simulink model "Energy Domain TDPC Q2"  (R2021b)
settings: Solver=ode4  StartTime=0.0  StopTime=20  FixedStep=0.0001  RelTol=1e-3
libraries: slpidlib x2
settings Model: Creator=rmkna  LastModifiedBy=rmkna

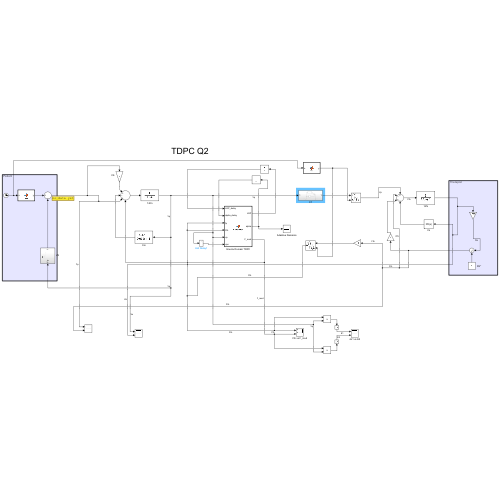
[thumbnail: Simulink's stored preview of the top-level diagram]
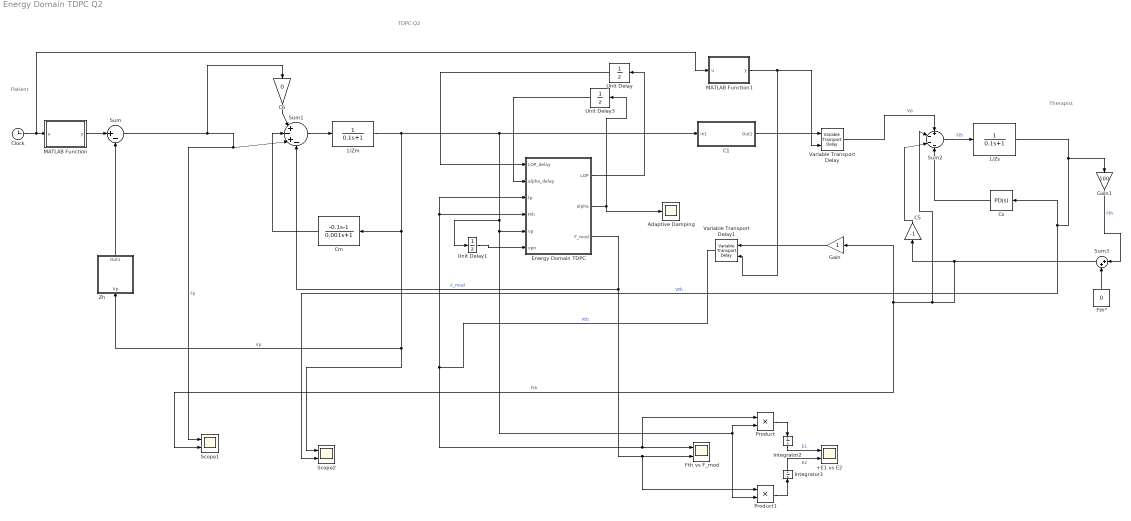
== system Energy Domain TDPC Q2 ==
  note: TDPC Q2
  note: Therapist
  note: Patient
  +E1 vs E2 : Scope  NumInputPorts=2
  1/Zm : TransferFcn  Denominator=[0.1 1]
  1/Zs : TransferFcn  Denominator=[0.1 1]
  Adaptive Damping : Scope
  C1 : Subsystem
  "C5 " : Gain  Gain=-1
  "C6 " : Gain  Gain=0
  Clock : Clock
  Cm : TransferFcn  Numerator=[-0.1 -1]  Denominator=[0.001 1]
  Cs : slpidlib/PID Controller  Controller=PD  Form=Parallel  TimeDomain=Continuous-time  UseExternalTs=off  SampleTime=-1  IntegratorMethod=Forward Euler  FilterMethod=Forward Euler  ControllerParametersSource=internal  P=1000  I=1  D=1  UseFilter=on  N=1000  TunerSelectOption=Transfer Function Based (PID Tuner App)  InitialConditionSource=internal  InitialConditionForIntegrator=0  InitialConditionForFilter=0  DifferentiatorICPrevScaledInput=0  ExternalReset=none  TrackingMode=off  Kt=1  LimitOutput=off  SatLimitsSource=internal  UpperSaturationLimit=inf  LowerSaturationLimit=-inf  LinearizeAsGain=on  AntiWindupMode=none  Kb=1  POutMin=[]  POutMax=[]  IOutMin=[]  IOutMax=[]  DOutMin=[]  DOutMax=[]  NOutMin=[]  NOutMax=[]  SumOutMin=[]  SumOutMax=[]  SaturationOutMin=[]  SaturationOutMax=[]  PParamMin=[]  PParamMax=[]  IParamMin=[]  IParamMax=[]  DParamMin=[]  DParamMax=[]  NParamMin=[]  NParamMax=[]  KbParamMin=[]  KbParamMax=[]  KtParamMin=[]  KtParamMax=[]  KbOutMin=[]  KbOutMax=[]  KtOutMin=[]  KtOutMax=[]  IntegratorOutMin=[]  IntegratorOutMax=[]  FilterOutMin=[]  FilterOutMax=[]  SumI1OutMin=[]  SumI1OutMax=[]  SumI2OutMin=[]  SumI2OutMax=[]  SumI3OutMin=[]  SumI3OutMax=[]  SumI4OutMin=[]  SumI4OutMax=[]  SumDOutMin=[]  SumDOutMax=[]  DifferentiatorOutMin=[]  DifferentiatorOutMax=[]  FilterDiffOutCoefMin=[]  FilterDiffOutCoefMax=[]  ReciprocalOutMin=[]  ReciprocalOutMax=[]  SumDenOutMin=[]  SumDenOutMax=[]  SumNumOutMin=[]  SumNumOutMax=[]  DivideOutMin=[]  DivideOutMax=[]  UdiffTsProdOutMin=[]  UdiffTsProdOutMax=[]  NTsProdOutMin=[]  NTsProdOutMax=[]  UintegralTsProdOutMin=[]  UintegralTsProdOutMax=[]  UngainTsProdOutMin=[]  UngainTsProdOutMax=[]  IntegratorContinuousStateAttributes=''  IntegratorStateMustResolveToSignalObject=off  IntegratorRTWStateStorageClass=Auto  FilterContinuousStateAttributes=''  FilterStateMustResolveToSignalObject=off  FilterRTWStateStorageClass=Auto  ParallelPVariant=InternalParameters  IdealPVariant=Disabled  IVariant=Disabled  DVariant=InternalParameters  IntegratorVariant=Disabled  SatVariant=Disabled  AWVariant=Disabled  PCopyVariant=Disabled  TRVariant=Disabled  FdbkBlocksVariant=Forward  IdealPFdbkVariant=Disabled  SatFdbkVariant=Disabled  DerivativeFilterVariant=ContFilter  NVariant=InternalParameters  NCopyVariant=Disabled  FilterICVariant=InternalICsFilter  IntegratorICVariant=Disabled  ExternalResetVariant=Disabled  TRSumVariant=Passthrough  SumFdbkVariant=Disabled  SumVariant=Sum_PD  TsampFilterVariant=InternalTs  TsampNgainVariant=Passthrough  TsampIntegralVariant=Disabled_SignalSpec  ExternalSaturationOutDataTypeStr=Inherit: Same as second input
  Energy Domain TDPC : MATLAB Function  TreatAsAtomicUnit=on
  Fth vs F_mod : Scope  NumInputPorts=2
  Fth* : Constant  Value=0  OutDataTypeStr=Inherit: Inherit via back propagation
  Gain : Gain
  Gain1 : Gain  Gain=100
  Integrator2 : Integrator
  Integrator3 : Integrator
  MATLAB Function : MATLAB Function  TreatAsAtomicUnit=on
  MATLAB Function1 : MATLAB Function  TreatAsAtomicUnit=on
  Product : Product
  Product1 : Product
  Scope1 : Scope  NumInputPorts=2
  Scope2 : Scope  NumInputPorts=2
  Sum : Sum  Inputs=|+-
  Sum1 : Sum  Inputs=|+-+-
  Sum2 : Sum  Inputs=+---
  Sum3 : Sum  Inputs=|++
  Unit Delay : UnitDelay  SampleTime=-1  HasFrameUpgradeWarning=on
  Unit Delay1 : UnitDelay  SampleTime=-1  HasFrameUpgradeWarning=on
  Unit Delay3 : UnitDelay  SampleTime=-1  HasFrameUpgradeWarning=on
  Variable Transport Delay : VariableTransportDelay
  Variable Transport Delay1 : VariableTransportDelay
  Zh : Subsystem
  wires:
  Integrator3/1 -> +E1 vs E2/2  "E2"
  "C5 "/1 -> Sum2/3
  Unit Delay3/1 -> Energy Domain TDPC/2(alpha_delay)
  1/Zs/1 -> Gain1/1, Cs/1, Scope2/2  "Vth"
  Variable Transport Delay/1 -> Sum2/1  "Vp"
  Product1/1 -> Integrator3/1
  Energy Domain TDPC/2(alpha) -> Adaptive Damping/1, Unit Delay3/1
  Unit Delay1/1 -> Energy Domain TDPC/6(vpn)
  Product/1 -> Integrator2/1
  C1/1(Out1) -> Variable Transport Delay/1
  Integrator2/1 -> +E1 vs E2/1  "E1"
  Gain/1 -> Variable Transport Delay1/1
  Energy Domain TDPC/3(F_mod) -> Product1/1, Fth vs F_mod/2, Sum1/4  "F_mod"
  Energy Domain TDPC/1(LOP) -> Unit Delay/1
  "C6 "/1 -> Sum1/1
  Cs/1 -> Sum2/4
  Variable Transport Delay1/1 -> Product/1, Fth vs F_mod/1, Energy Domain TDPC/3(fp), Energy Domain TDPC/4(Fth)  "Fth"
  Sum/1 -> "C6 "/1, Scope1/1, Sum1/3  "Fp"
  MATLAB Function1/1(y) -> Variable Transport Delay1/2, Variable Transport Delay/2
  1/Zm/1 -> Scope2/1, Zh/1(Vp), Cm/1, Energy Domain TDPC/5(vp), Product1/2, Product/2, Unit Delay1/1, C1/1(In1)  "Vp"
  Unit Delay/1 -> Energy Domain TDPC/1(LOP_delay)
  Sum3/1 -> Sum2/2, Gain/1, Scope1/2, "C5 "/1  "Fth"
  Sum2/1 -> 1/Zs/1  "Fth"
  Fth*/1 -> Sum3/2
  Sum1/1 -> 1/Zm/1
  Cm/1 -> Sum1/2
  Gain1/1 -> Sum3/1  "Fth"
  Zh/1(Out1) -> Sum/2
  MATLAB Function/1(y) -> Sum/1
  Clock/1 -> MATLAB Function1/1(u), MATLAB Function/1(u)

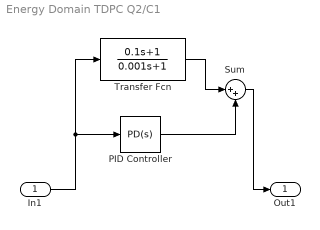
== system Energy Domain TDPC Q2/C1 ==
  In1 : Inport
  PID Controller : slpidlib/PID Controller  Controller=PD  Form=Parallel  TimeDomain=Continuous-time  UseExternalTs=off  SampleTime=-1  IntegratorMethod=Forward Euler  FilterMethod=Forward Euler  ControllerParametersSource=internal  P=1000  I=1  D=1  UseFilter=on  N=1000  TunerSelectOption=Transfer Function Based (PID Tuner App)  InitialConditionSource=internal  InitialConditionForIntegrator=0  InitialConditionForFilter=0  DifferentiatorICPrevScaledInput=0  ExternalReset=none  TrackingMode=off  Kt=1  LimitOutput=off  SatLimitsSource=internal  UpperSaturationLimit=inf  LowerSaturationLimit=-inf  LinearizeAsGain=on  AntiWindupMode=none  Kb=1  POutMin=[]  POutMax=[]  IOutMin=[]  IOutMax=[]  DOutMin=[]  DOutMax=[]  NOutMin=[]  NOutMax=[]  SumOutMin=[]  SumOutMax=[]  SaturationOutMin=[]  SaturationOutMax=[]  PParamMin=[]  PParamMax=[]  IParamMin=[]  IParamMax=[]  DParamMin=[]  DParamMax=[]  NParamMin=[]  NParamMax=[]  KbParamMin=[]  KbParamMax=[]  KtParamMin=[]  KtParamMax=[]  KbOutMin=[]  KbOutMax=[]  KtOutMin=[]  KtOutMax=[]  IntegratorOutMin=[]  IntegratorOutMax=[]  FilterOutMin=[]  FilterOutMax=[]  SumI1OutMin=[]  SumI1OutMax=[]  SumI2OutMin=[]  SumI2OutMax=[]  SumI3OutMin=[]  SumI3OutMax=[]  SumI4OutMin=[]  SumI4OutMax=[]  SumDOutMin=[]  SumDOutMax=[]  DifferentiatorOutMin=[]  DifferentiatorOutMax=[]  FilterDiffOutCoefMin=[]  FilterDiffOutCoefMax=[]  ReciprocalOutMin=[]  ReciprocalOutMax=[]  SumDenOutMin=[]  SumDenOutMax=[]  SumNumOutMin=[]  SumNumOutMax=[]  DivideOutMin=[]  DivideOutMax=[]  UdiffTsProdOutMin=[]  UdiffTsProdOutMax=[]  NTsProdOutMin=[]  NTsProdOutMax=[]  UintegralTsProdOutMin=[]  UintegralTsProdOutMax=[]  UngainTsProdOutMin=[]  UngainTsProdOutMax=[]  IntegratorContinuousStateAttributes=''  IntegratorStateMustResolveToSignalObject=off  IntegratorRTWStateStorageClass=Auto  FilterContinuousStateAttributes=''  FilterStateMustResolveToSignalObject=off  FilterRTWStateStorageClass=Auto  ParallelPVariant=InternalParameters  IdealPVariant=Disabled  IVariant=Disabled  DVariant=InternalParameters  IntegratorVariant=Disabled  SatVariant=Disabled  AWVariant=Disabled  PCopyVariant=Disabled  TRVariant=Disabled  FdbkBlocksVariant=Forward  IdealPFdbkVariant=Disabled  SatFdbkVariant=Disabled  DerivativeFilterVariant=ContFilter  NVariant=InternalParameters  NCopyVariant=Disabled  FilterICVariant=InternalICsFilter  IntegratorICVariant=Disabled  ExternalResetVariant=Disabled  TRSumVariant=Passthrough  SumFdbkVariant=Disabled  SumVariant=Sum_PD  TsampFilterVariant=InternalTs  TsampNgainVariant=Passthrough  TsampIntegralVariant=Disabled_SignalSpec  ExternalSaturationOutDataTypeStr=Inherit: Same as second input
  Sum : Sum  Inputs=|++
  Transfer Fcn : TransferFcn  Numerator=[0.1 1]  Denominator=[0.001 1]
  Out1 : Outport
  wires:
  In1/1 -> PID Controller/1, Transfer Fcn/1
  Transfer Fcn/1 -> Sum/1
  PID Controller/1 -> Sum/2
  Sum/1 -> Out1/1

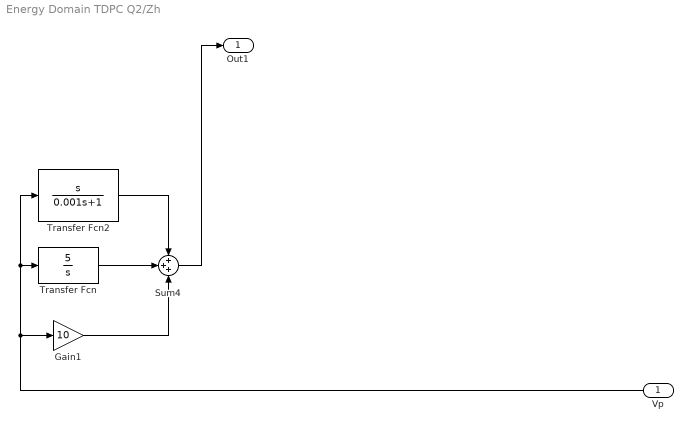
== system Energy Domain TDPC Q2/Zh ==
  Vp : Inport
  Gain1 : Gain  Gain=10
  Sum4 : Sum  Inputs=3
  Transfer Fcn : TransferFcn  Numerator=[5]  Denominator=[1 0]
  Transfer Fcn2 : TransferFcn  Numerator=[1 0]  Denominator=[0.001 1]
  Out1 : Outport
  wires:
  Vp/1 -> Gain1/1, Transfer Fcn/1, Transfer Fcn2/1
  Sum4/1 -> Out1/1
  Transfer Fcn/1 -> Sum4/2
  Transfer Fcn2/1 -> Sum4/1
  Gain1/1 -> Sum4/3

== matlab function Energy Domain TDPC Q2/MATLAB Function1 ==
  data: u input; y output
function y = fcn(u)

y = 0.1+0.02*cos(12*u);

== matlab function Energy Domain TDPC Q2/Energy Domain TDPC ==
  data: LOP_delay input; alpha_delay input; LOP output; alpha output; fp input; Fth input; F_mod output; vp input; vpn input
function [LOP,alpha, F_mod] = Stabilizer(LOP_delay,alpha_delay,fp,Fth,vp,vpn)

PL = (fp'*vp);
in2 = (alpha_delay*(vpn')*vpn);
LOP = LOP_delay+(0.001*(PL+in2));

if LOP>=0
    alpha = 0;
else 
    alpha=(-LOP)/(0.001*(vp')*vp)+0.00001;
end

F_mod= Fth+(alpha*vp)+0.00001;

== matlab function Energy Domain TDPC Q2/MATLAB Function ==
  data: u input; y output
function y = fcn(u)

y = sin(5*u)+ cos(8*u);
